simulink library "Lib_Controller"  (R2019b)
settings: Solver=VariableStepAuto  StartTime=0.0  StopTime=10.0  RelTol=1e-3
undefined symbols (not defined in the file): apollo_control_timeout, controller_max_time_diff, controller_params, DiscIntNeverNeededParam, max_acceleration_comfort, max_deceleration_comfort, max_long_jerk_comfort, max_steering_speed_comfort, min_long_jerk_comfort, steering_angle_range_rad_to_steering_wheel_angle_range_deg_gain, switch_steering_feedback, switch_velocity_feedback
libraries: Lib_ReferencePointCalculation x1, simulink x1
settings Model: Creator=esterle  LastModifiedBy=kessler
settings DataIOCC: ReturnWorkspaceOutputs=off
settings DebuggingCC: ArithmeticOperatorsInVariantConditions=warning
settings SFSimCC: SimUseLocalCustomCode=off  CustomCodeUndefinedFunction=UseInterfaceOnly
settings RTWCC: RTWUseLocalCustomCode=off

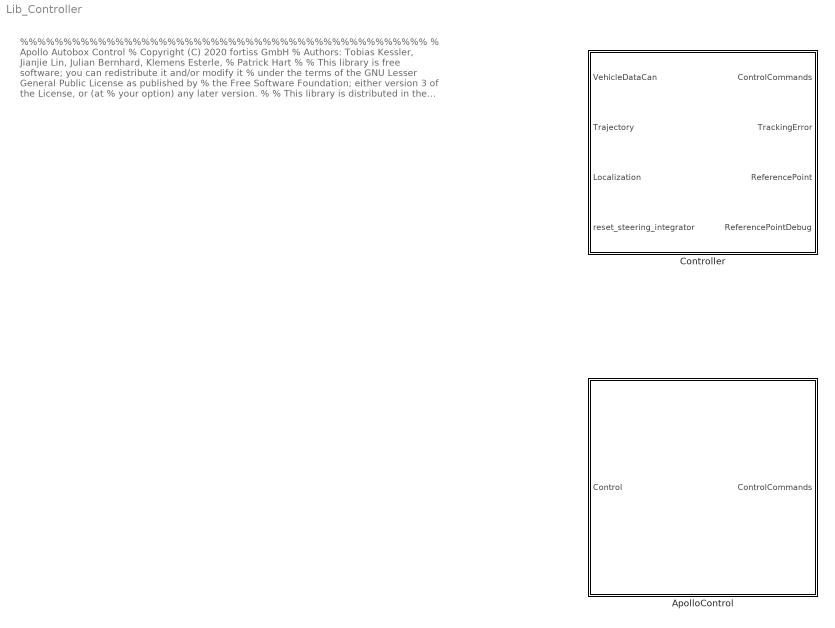
== system Lib_Controller ==
  note: %%%%%%%%%%%%%%%%%%%%%%%%%%%%%%%%%%%%%%%%%%%%%%%
      | % Apollo Autobox Control
      | % Copyright (C) 2020 fortiss GmbH
      | % Authors: Tobias Kessler, Jianjie Lin, Julian Bernhard, Klemens Esterle,
      | % Patrick Hart
      | %
      | % This library is free software; you can redistribute it and/or modify it
      | % under the terms of the GNU Lesser General Public License as published by
      | % the Free Software Foundation; either version 3 of the License, or (at
      | % your option) any later version.
      | %
      | % This library is distributed in the hope that it will be useful, but
      | % WITHOUT ANY WARRANTY; without even the implied warranty of
      | % MERCHANTABILITY or FITNESS FOR A PARTICULAR PURPOSE. See the GNU Lesser
      | % General Public License for more details.
      | %
      | % You should have received a copy of the GNU Lesser General Public License
      | % along with this library; if not, write to the Free Software Foundation,
      | % Inc., 51 Franklin Street, Fifth Floor, Boston, MA 02110-1301, USA.
      | %%%%%%%%%%%%%%%%%%%%%%%%%%%%%%%%%%%%%%%%%%%%%%%
  ApolloControl : Subsystem
  Controller : Subsystem

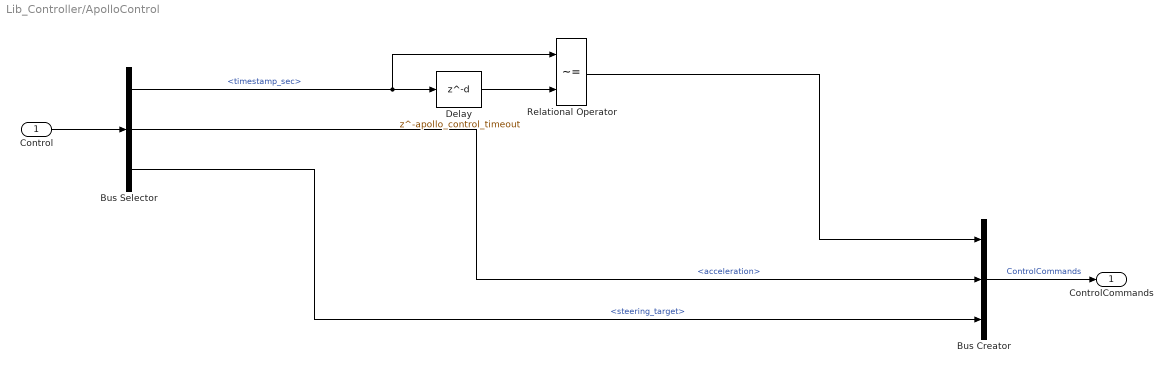
== system Lib_Controller/ApolloControl ==
  Control : Inport
  Bus Creator : BusCreator  Inputs=3  OutDataTypeStr=Bus: ControlCommands
      settings: InheritFromInputs=off
  Bus Selector : BusSelector  OutputSignals=timestamp_sec,acceleration,steering_target
  Delay : Delay  DelayLength=apollo_control_timeout
  Relational Operator : RelationalOperator  Operator=~=  OutDataTypeStr=boolean  RndMeth=Simplest
  ControlCommands : Outport
  wires:
  Bus Creator/1 -> ControlCommands/1  "ControlCommands"
  Control/1 -> Bus Selector/1
  Bus Selector/2 -> Bus Creator/2  "<acceleration>"
  Bus Selector/3 -> Bus Creator/3  "<steering_target>"
  Bus Selector/1 -> Relational Operator/1, Delay/1  "<timestamp_sec>"
  Delay/1 -> Relational Operator/2
  Relational Operator/1 -> Bus Creator/1

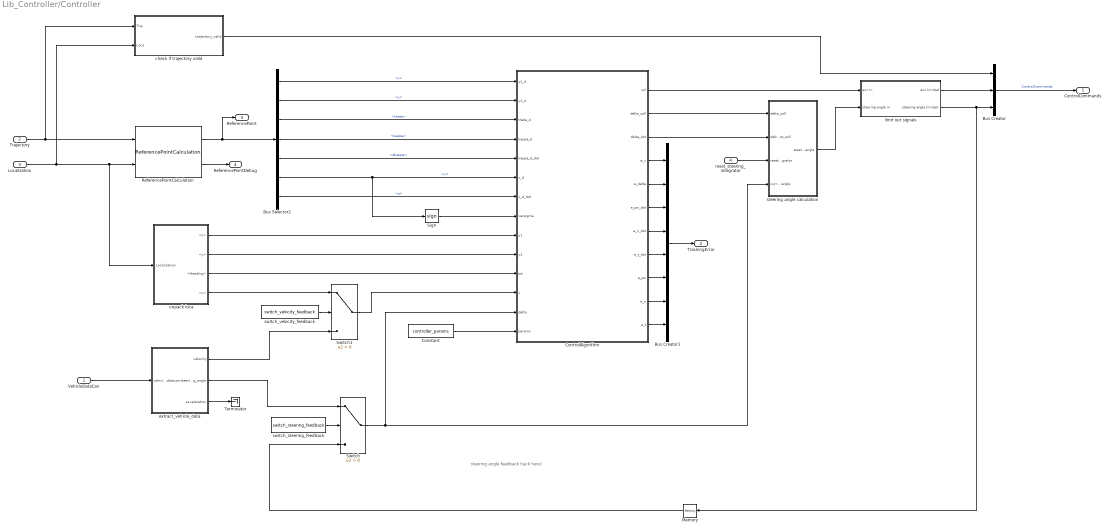
== system Lib_Controller/Controller ==
  note: steering angle feedback hack here!
  VehicleDataCan : Inport  OutDataTypeStr=Bus: vehicle_data_can_bus  BusOutputAsStruct=on
  Trajectory : Inport  Port=2  OutDataTypeStr=Bus: ControlTrajectory  BusOutputAsStruct=on
  Localization : Inport  Port=3  OutDataTypeStr=Bus: LocalizationToAutobox  BusOutputAsStruct=on
  reset_steering_integrator : Inport  Port=4
  Bus Creator : BusCreator  Inputs=3  OutDataTypeStr=Bus: ControlCommands
      settings: InheritFromInputs=off
  Bus Creator1 : BusCreator  Inputs=8  OutDataTypeStr=Bus: TrackingError  NonVirtualBus=on
  Bus Selector2 : BusSelector  OutputSignals=x,y,theta,kappa,dkappa,v,a
  Constant : Constant  Value=controller_params  OutDataTypeStr=Bus: ControllerParams
  ControlAlgorithm : MATLAB Function  TreatAsAtomicUnit=on
  Memory : Memory
  ReferencePointCalculation : Lib_ReferencePointCalculation/ReferencePointCalculation
  Sign : Signum
  Switch : Switch  Criteria=u2 > Threshold
  Switch1 : Switch  Criteria=u2 > Threshold
  Terminator : Terminator
  check if trajectory valid : Subsystem
  extract_vehicle_data : Subsystem
  limit out signals : Subsystem
  steering angle calculation : Subsystem
  switch_steering_feedback : Constant  Value=switch_steering_feedback
  switch_velocity_feedback : Constant  Value=switch_velocity_feedback
  unpack loca : Subsystem
  ControlCommands : Outport  OutDataTypeStr=Bus: ControlCommands  VectorParamsAs1DForOutWhenUnconnected=off
  TrackingError : Outport  Port=2  OutDataTypeStr=Bus: TrackingError  VectorParamsAs1DForOutWhenUnconnected=off
  ReferencePoint : Outport  Port=3  OutDataTypeStr=Bus: TrajectoryPoint  VectorParamsAs1DForOutWhenUnconnected=off
  ReferencePointDebug : Outport  Port=4  VectorParamsAs1DForOutWhenUnconnected=off
  wires:
  check if trajectory valid/1(trajectory_valid) -> Bus Creator/1
  Switch1/1 -> ControlAlgorithm/12(v)
  extract_vehicle_data/1(velocity) -> Switch1/3
  switch_velocity_feedback/1 -> Switch1/2
  extract_vehicle_data/2(steering_angle) -> Switch/1
  switch_steering_feedback/1 -> Switch/2
  Memory/1 -> Switch/3
  ReferencePointCalculation/2 -> ReferencePointDebug/1
  unpack loca/3(<Heading>) -> ControlAlgorithm/11(psi)
  unpack loca/2(<y>) -> ControlAlgorithm/10(y2)
  unpack loca/1(<x>) -> ControlAlgorithm/9(y1)
  extract_vehicle_data/3(acceleration) -> Terminator/1
  VehicleDataCan/1 -> extract_vehicle_data/1(vehicledatacan)
  unpack loca/4(<v>) -> Switch1/1
  Switch/1 -> steering angle calculation/4(current_steering angle), ControlAlgorithm/13(delta)
  limit out signals/2(steering angle limited) -> Bus Creator/3, Memory/1
  limit out signals/1(acc limited) -> Bus Creator/2
  steering angle calculation/1(steering_angle) -> limit out signals/2(steering angle in)
  ControlAlgorithm/1(w2) -> limit out signals/1(acc in)
  reset_steering_integrator/1 -> steering angle calculation/3(reset_steering_integrator)
  ControlAlgorithm/3(delta_dot) -> steering angle calculation/2(delta_dot_soll)
  ControlAlgorithm/2(delta_soll) -> steering angle calculation/1(delta_soll)
  Sign/1 -> ControlAlgorithm/8(varsigma)
  ReferencePointCalculation/1 -> ReferencePoint/1, Bus Selector2/1
  Trajectory/1 -> ReferencePointCalculation/1, check if trajectory valid/1(Traj)
  Bus Creator/1 -> ControlCommands/1  "ControlCommands"
  Bus Selector2/2 -> ControlAlgorithm/2(y2_d)  "<y>"
  Bus Selector2/4 -> ControlAlgorithm/4(kappa_d)  "<kappa>"
  Bus Selector2/3 -> ControlAlgorithm/3(theta_d)  "<theta>"
  Bus Selector2/5 -> ControlAlgorithm/5(kappa_d_dot)  "<dkappa>"
  Bus Selector2/7 -> ControlAlgorithm/7(v_d_dot)  "<a>"
  Bus Selector2/1 -> ControlAlgorithm/1(y1_d)  "<x>"
  Localization/1 -> ReferencePointCalculation/2, unpack loca/1(Localization), check if trajectory valid/2(Loca)
  Bus Creator1/1 -> TrackingError/1
  Bus Selector2/6 -> ControlAlgorithm/6(v_d), Sign/1  "<v>"
  Constant/1 -> ControlAlgorithm/14(params)
  ControlAlgorithm/4(e_v) -> Bus Creator1/1
  ControlAlgorithm/5(e_delta) -> Bus Creator1/2
  ControlAlgorithm/6(e_psi_dot) -> Bus Creator1/3
  ControlAlgorithm/7(e_n_dot) -> Bus Creator1/4
  ControlAlgorithm/8(e_t_dot) -> Bus Creator1/5
  ControlAlgorithm/9(e_psi) -> Bus Creator1/6
  ControlAlgorithm/10(e_n) -> Bus Creator1/7
  ControlAlgorithm/11(e_t) -> Bus Creator1/8

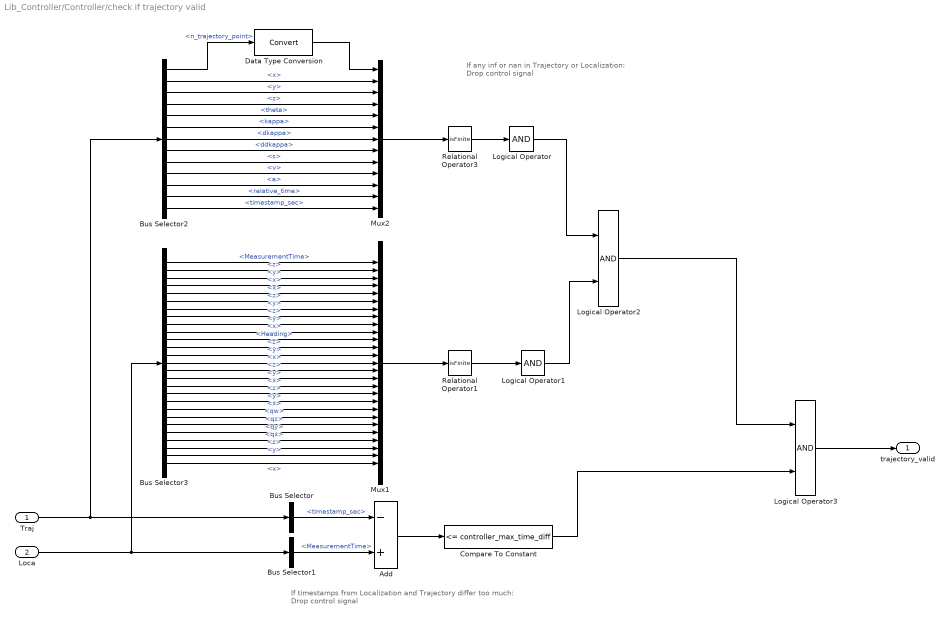
== system Lib_Controller/Controller/check if trajectory valid ==
  note: If timestamps from Localization and Trajectory differ too much:
      | Drop control signal
  note: If any inf or nan in Trajectory or Localization:
      | Drop control signal
  Traj : Inport
  Loca : Inport  Port=2
  Add : Sum  Inputs=-+
  Bus Selector : BusSelector  OutputSignals=timestamp_sec
  Bus Selector1 : BusSelector  OutputSignals=MeasurementTime
  Bus Selector2 : BusSelector  OutputSignals=n_trajectory_point,x,y,z,theta,kappa,dkappa,ddkappa,s,v,a,relative_time,timestamp_sec
  Bus Selector3 : BusSelector  OutputSignals=MeasurementTime,Pose.EulerAngles.z,Pose.EulerAngles.y,Pose.EulerAngles.x,Pose.AngularVelocityVrf.x,Pose.AngularVelocityVrf.z,Pose.AngularVelocityVrf.y,Pose.LinearAccelerationVrf.z,Pose.LinearAccelerationVrf.y,Pose.LinearAccelerationVrf.x,Pose.Heading,Pose.AngularVelocity.z,Pose.AngularVelocity.y,Pose.AngularVelocity.x,Pose.LinearAcceleration.z,Pose.LinearAcceleration.y,Pose.LinearAcceleration.x,Pose.LinearVelocity.z,Pose.LinearVelocity.y,Pose.LinearVelocity.x,Pose.Orientation.qw,Pose.Orientation.qz,Pose.Orientation.qy,Pose.Orientation.qx,Pose.Position.z,Pose.Position.y,Pose.Position.x
  Compare To Constant : simulink/Logic and Bit Operations/Compare To Constant  relop=<=  const=controller_max_time_diff  OutDataTypeStr=boolean
  Data Type Conversion : DataTypeConversion
  Logical Operator : Logic  Inputs=1  AllPortsSameDT=off  OutDataTypeStr=boolean
  Logical Operator1 : Logic  Inputs=1  AllPortsSameDT=off  OutDataTypeStr=boolean
  Logical Operator2 : Logic  AllPortsSameDT=off  OutDataTypeStr=boolean
  Logical Operator3 : Logic  AllPortsSameDT=off  OutDataTypeStr=boolean
  Mux1 : Mux  Inputs=27
  Mux2 : Mux  Inputs=13
  Relational Operator1 : RelationalOperator  Operator=isFinite  OutDataTypeStr=boolean  RndMeth=Simplest
  Relational Operator3 : RelationalOperator  Operator=isFinite  OutDataTypeStr=boolean  RndMeth=Simplest
  trajectory_valid : Outport  VectorParamsAs1DForOutWhenUnconnected=off
  wires:
  Data Type Conversion/1 -> Mux2/1
  Bus Selector3/27 -> Mux1/27  "<x>"
  Bus Selector3/26 -> Mux1/26  "<y>"
  Bus Selector3/25 -> Mux1/25  "<z>"
  Bus Selector3/24 -> Mux1/24  "<qx>"
  Bus Selector3/23 -> Mux1/23  "<qy>"
  Bus Selector3/22 -> Mux1/22  "<qz>"
  Bus Selector3/21 -> Mux1/21  "<qw>"
  Bus Selector3/20 -> Mux1/20  "<x>"
  Bus Selector3/19 -> Mux1/19  "<y>"
  Bus Selector3/18 -> Mux1/18  "<z>"
  Bus Selector3/17 -> Mux1/17  "<x>"
  Bus Selector3/16 -> Mux1/16  "<y>"
  Bus Selector3/15 -> Mux1/15  "<z>"
  Bus Selector3/14 -> Mux1/14  "<x>"
  Bus Selector3/13 -> Mux1/13  "<y>"
  Bus Selector3/12 -> Mux1/12  "<z>"
  Bus Selector3/11 -> Mux1/11  "<Heading>"
  Bus Selector3/1 -> Mux1/1  "<MeasurementTime>"
  Bus Selector3/10 -> Mux1/10  "<x>"
  Bus Selector3/2 -> Mux1/2  "<z>"
  Bus Selector3/9 -> Mux1/9  "<y>"
  Bus Selector3/3 -> Mux1/3  "<y>"
  Bus Selector3/8 -> Mux1/8  "<z>"
  Bus Selector3/4 -> Mux1/4  "<x>"
  Bus Selector3/7 -> Mux1/7  "<y>"
  Bus Selector3/5 -> Mux1/5  "<x>"
  Bus Selector3/6 -> Mux1/6  "<z>"
  Bus Selector2/13 -> Mux2/13  "<timestamp_sec>"
  Bus Selector2/12 -> Mux2/12  "<relative_time>"
  Bus Selector2/11 -> Mux2/11  "<a>"
  Bus Selector2/1 -> Data Type Conversion/1  "<n_trajectory_point>"
  Bus Selector2/2 -> Mux2/2  "<x>"
  Bus Selector2/3 -> Mux2/3  "<y>"
  Bus Selector2/4 -> Mux2/4  "<z>"
  Bus Selector2/5 -> Mux2/5  "<theta>"
  Bus Selector2/10 -> Mux2/10  "<v>"
  Bus Selector2/6 -> Mux2/6  "<kappa>"
  Bus Selector2/9 -> Mux2/9  "<s>"
  Bus Selector2/7 -> Mux2/7  "<dkappa>"
  Bus Selector2/8 -> Mux2/8  "<ddkappa>"
  Mux1/1 -> Relational Operator1/1
  Mux2/1 -> Relational Operator3/1
  Compare To Constant/1 -> Logical Operator3/2
  Relational Operator3/1 -> Logical Operator/1
  Relational Operator1/1 -> Logical Operator1/1
  Loca/1 -> Bus Selector3/1, Bus Selector1/1
  Traj/1 -> Bus Selector/1, Bus Selector2/1
  Logical Operator2/1 -> Logical Operator3/1
  Logical Operator1/1 -> Logical Operator2/2
  Logical Operator/1 -> Logical Operator2/1
  Logical Operator3/1 -> trajectory_valid/1
  Add/1 -> Compare To Constant/1
  Bus Selector1/1 -> Add/2  "<MeasurementTime>"
  Bus Selector/1 -> Add/1  "<timestamp_sec>"

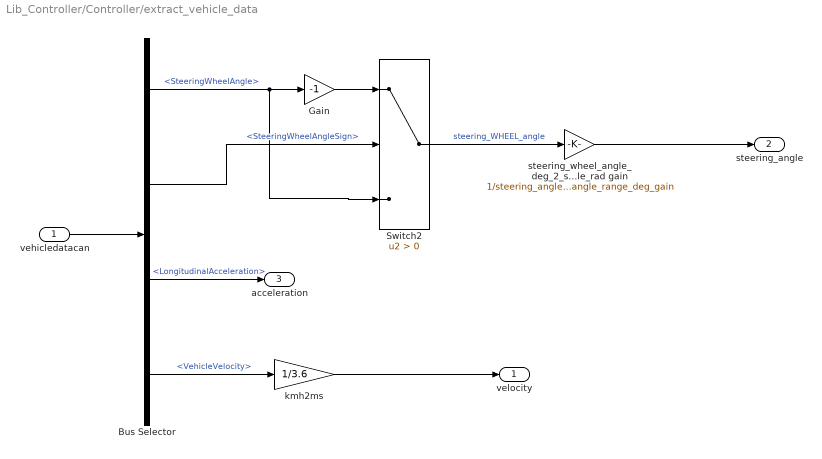
== system Lib_Controller/Controller/extract_vehicle_data ==
  vehicledatacan : Inport
  Bus Selector : BusSelector  OutputSignals=Steering.SteeringWheelAngle,Steering.SteeringWheelAngleSign,Motion.LongitudinalAcceleration,Motion.VehicleVelocity
  Gain : Gain  Gain=-1
  Switch2 : Switch  Criteria=u2 > Threshold
  kmh2ms : Gain  Gain=1/3.6
  steering_wheel_angle_deg_2_steering_angle_rad gain : Gain  Gain=1/steering_angle_range_rad_to_steering_wheel_angle_range_deg_gain
  velocity : Outport  VectorParamsAs1DForOutWhenUnconnected=off
  steering_angle : Outport  Port=2  VectorParamsAs1DForOutWhenUnconnected=off
  acceleration : Outport  Port=3  VectorParamsAs1DForOutWhenUnconnected=off
  wires:
  steering_wheel_angle_deg_2_steering_angle_rad gain/1 -> steering_angle/1
  Bus Selector/1 -> Gain/1, Switch2/3  "<SteeringWheelAngle>"
  Gain/1 -> Switch2/1
  Bus Selector/2 -> Switch2/2  "<SteeringWheelAngleSign>"
  kmh2ms/1 -> velocity/1
  Bus Selector/4 -> kmh2ms/1  "<VehicleVelocity>"
  Bus Selector/3 -> acceleration/1  "<LongitudinalAcceleration>"
  Switch2/1 -> steering_wheel_angle_deg_2_steering_angle_rad gain/1  "steering_WHEEL_angle"
  vehicledatacan/1 -> Bus Selector/1

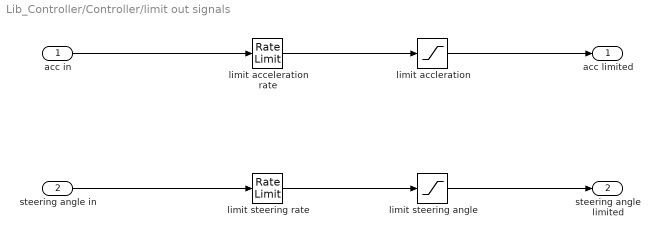
== system Lib_Controller/Controller/limit out signals ==
  acc in : Inport
  steering angle in : Inport  Port=2
  limit acceleration rate : RateLimiter  RisingSlewLimit=max_long_jerk_comfort  FallingSlewLimit=min_long_jerk_comfort  SampleTimeMode=inherited
  limit accleration : Saturate  UpperLimit=max_acceleration_comfort  LowerLimit=max_deceleration_comfort
  limit steering angle : Saturate  UpperLimit=0.61  LowerLimit=-0.61
  limit steering rate : RateLimiter  RisingSlewLimit=max_steering_speed_comfort  FallingSlewLimit=-max_steering_speed_comfort  SampleTimeMode=inherited
  acc limited : Outport  VectorParamsAs1DForOutWhenUnconnected=off
  steering angle limited : Outport  Port=2  VectorParamsAs1DForOutWhenUnconnected=off
  wires:
  limit acceleration rate/1 -> limit accleration/1
  limit steering rate/1 -> limit steering angle/1
  limit accleration/1 -> acc limited/1
  limit steering angle/1 -> steering angle limited/1
  steering angle in/1 -> limit steering rate/1
  acc in/1 -> limit acceleration rate/1

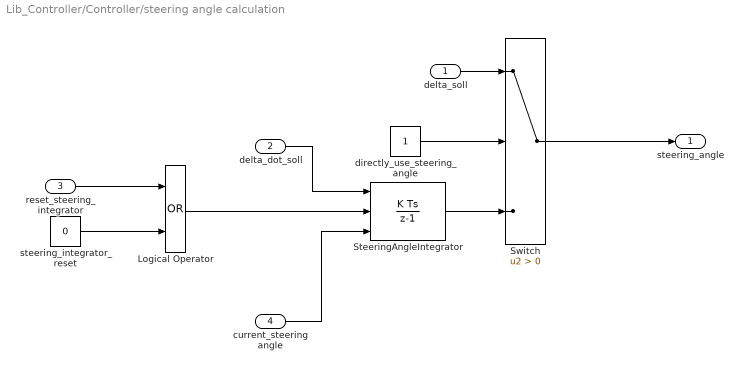
== system Lib_Controller/Controller/steering angle calculation ==
  delta_soll : Inport
  delta_dot_soll : Inport  Port=2
  reset_steering_integrator : Inport  Port=3
  current_steering angle : Inport  Port=4
  Logical Operator : Logic  Operator=OR  AllPortsSameDT=off  OutDataTypeStr=boolean
  SteeringAngleIntegrator : DiscreteIntegrator  ExternalReset=rising  InitialConditionSource=external  SampleTime=-1  ICPrevOutput=DiscIntNeverNeededParam  ICPrevScaledInput=DiscIntNeverNeededParam
  Switch : Switch  Criteria=u2 > Threshold
  directly_use_steering_angle : Constant
  steering_integrator_reset : Constant  Value=0  OutDataTypeStr=boolean
  steering_angle : Outport  VectorParamsAs1DForOutWhenUnconnected=off
  wires:
  Logical Operator/1 -> SteeringAngleIntegrator/2
  steering_integrator_reset/1 -> Logical Operator/2
  reset_steering_integrator/1 -> Logical Operator/1
  SteeringAngleIntegrator/1 -> Switch/3
  directly_use_steering_angle/1 -> Switch/2
  current_steering angle/1 -> SteeringAngleIntegrator/3
  delta_soll/1 -> Switch/1
  delta_dot_soll/1 -> SteeringAngleIntegrator/1
  Switch/1 -> steering_angle/1

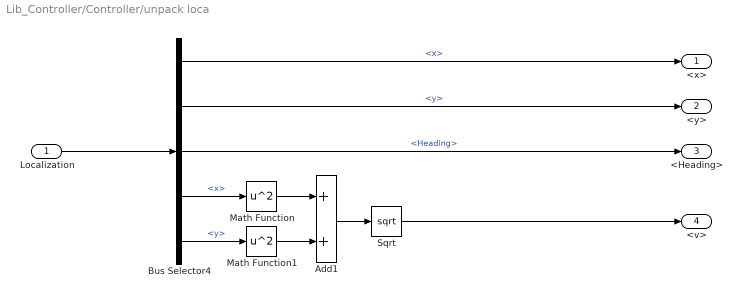
== system Lib_Controller/Controller/unpack loca ==
  Localization : Inport
  Add1 : Sum
  Bus Selector4 : BusSelector  OutputSignals=Pose.Position.x,Pose.Position.y,Pose.Heading,Pose.LinearVelocity.x,Pose.LinearVelocity.y
  Math Function : Math  Operator=square  SaturateOnIntegerOverflow=on
  Math Function1 : Math  Operator=square  SaturateOnIntegerOverflow=on
  Sqrt : Sqrt  SaturateOnIntegerOverflow=on
  <x> : Outport  VectorParamsAs1DForOutWhenUnconnected=off
  <y> : Outport  Port=2  VectorParamsAs1DForOutWhenUnconnected=off
  <Heading> : Outport  Port=3  VectorParamsAs1DForOutWhenUnconnected=off
  <v> : Outport  Port=4  VectorParamsAs1DForOutWhenUnconnected=off
  wires:
  Math Function1/1 -> Add1/2
  Bus Selector4/5 -> Math Function1/1  "<y>"
  Localization/1 -> Bus Selector4/1
  Sqrt/1 -> <v>/1
  Math Function/1 -> Add1/1
  Bus Selector4/4 -> Math Function/1  "<x>"
  Add1/1 -> Sqrt/1
  Bus Selector4/3 -> <Heading>/1  "<Heading>"
  Bus Selector4/1 -> <x>/1  "<x>"
  Bus Selector4/2 -> <y>/1  "<y>"

== matlab function Lib_Controller/Controller/ControlAlgorithm ==
  data: w2 output; delta_soll output; y1_d input; y2_d input; theta_d input; kappa_d input; kappa_d_dot input; v_d input; v_d_dot input; varsigma input; y1 input; y2 input; psi input; v input; delta input; params input; delta_dot output; e_v output; e_delta output; e_psi_dot output; e_n_dot output; e_t_dot output; e_psi output; e_n output; e_t output
function [w2, delta_soll, delta_dot, e_v, e_delta, e_psi_dot, e_n_dot, e_t_dot, e_psi, e_n, e_t] = kin_tracking_with_orientation_stab( ...
y1_d, y2_d, theta_d, kappa_d, kappa_d_dot, v_d, v_d_dot, varsigma, ...
y1, y2, psi, v, delta,...
params)

l_v = params.l_v;
l_h = params.l_h;
m = params.m;
J = params.J;
k1 = params.k1;
k2 = params.k2;
k3 = params.k3;
k4 = params.k4;

% y1_d, ..., varsigma: desired values in rear axle coordinates
% y1, ..., delta: measured states
% l_v, ..., gam: vehicular parameters
% k1, ..., k4: control design parameters

l = l_v + l_h; % wheel base
gam = 0;


% State transformations
e_t = ( y1-y1_d ) * cos(theta_d) + ( y2-y2_d ) * sin(theta_d); % (4.9)
e_n = ( y1-y1_d ) * (-sin(theta_d)) + ( y2-y2_d ) * cos(theta_d); % (4.9)
e_psi = ( psi - theta_d ); 
% Normalize to -pi..pi (4.9)
while(e_psi > pi)
    e_psi = e_psi - 2* pi;
end
while (e_psi < -pi)
    e_psi = e_psi + 2* pi;
end
    


kappa_delta = tan(delta)/l; % (4.9)

% Transformed time derivatives
e_t_dot = v*cos(e_psi) - v_d*( 1- kappa_d*e_n ); % (4.10a)
e_n_dot = v*sin(e_psi) - v_d*kappa_d*e_t; % (4.10b)
e_psi_dot = v*kappa_delta - v_d*kappa_d; % (4.10c)


% Taylor approximations for control law
cos_approx = -1/2*e_psi + 1/24*e_psi^3 - 1/720*e_psi^5; % (A.10)
sin_approx = 1 - 1/6*e_psi^2 + 1/120*e_psi^4 - 1/5040*e_psi^6; % (A.11)
dcos_approx = -0.5 + 1/8*e_psi^2 - 1/144*e_psi^4 + 1/5760*e_psi^6; % (A.12)
dsin_approx = -1/3*e_psi + 1/30*e_psi^3 - 1/840*e_psi^5; % (A.13)

% Fictitious and virtual control laws
xi1 = kappa_d - k1*( e_t*cos_approx + e_n*sin_approx ) - varsigma*k2*e_psi; % (4.11)
e_v = v - v_d;
w2 = v_d_dot - k1*e_t - k3 * e_v + varsigma*k2*e_psi^2 - e_psi * kappa_d; % (4.12)

% Back-stepping
xi1_dot = kappa_d_dot - k1*( e_t_dot*cos_approx ...
+ e_t*e_psi_dot*dcos_approx + e_n_dot*sin_approx ...
+ e_n*e_psi_dot*dsin_approx) - varsigma*k2*e_psi_dot; % (4.18)
e_delta = kappa_delta - xi1; % (4.16)
w1 = -e_psi*v + xi1_dot - k4*e_delta; % (4.17)


% Lateral input resubstitution
u1 = l*w1*cos(delta)^2; % (4.15)
delta_soll = atan(xi1*l);


% Longitudinal input resubstitution
M = ( m*l_h^2 + J ) / l^2;
u2 = 1/(1+gam*(1/cos(delta) - 1))*( w2*( m + M*tan(delta)^2 ) ...
+ 2*M*v*tan(delta)/cos(delta)^2*u1 ); % (4.7)

% Output results
delta_dot = u1;
F_l = u2;

end
